simulink model "Querdynamikmodell"  (R2018b)
settings: Solver=VariableStepAuto  StartTime=0.0  StopTime=10.0  RelTol=1e-3
model workspace (MAT data in the model file):
  chStern = 20.5517740291
  controllerActive = 0
  cvStern = 205.517740291
  deltaH = [0 0.02 0.04 0.06 0.08 0.1 0.12 0.14 0.16 0.18 0.2 0.22 0.24 0.26 0.28 0.3 0.32 0.34 0.36 0.38 0.4 0.42 0.44 0.46 0.48 0.5 0.52 0.54 0.56 0.58 0.6 0.62 0.64 0.66 0.68 0.7 0.72 0.74 0.76 0.78 0.8 0.82 0.84 0.86 0.88 0.9 0.92 0.94 0.96 0.98 1 1.02 1.04 1.06 1.08 1.1 1.12 1.14 1.16 1.18 1.2 1.22 1.24 1.26 1.28 1.3 1.32 1.34 1.36 1.38 1.4 1.42 1.44 1.46 1.48 1.5 1.52 1.54 1.56 1.58 1.6 1.62 1.64 1.66 1.68 1.7 1.72 1.74 1.76 1.78 1.8 1.82 1.84 1.86 1.88 1.9 1.92 1.94 1.96 1.98 2 2.02 2.04 2.06 2.08 2.1 2.12 2.14 2.16 2.18 2.2 2.22 2.24 2.26 2.28 2.3 2.32 2.34 2.36 2.38 2.4 2.42 2.44 2.46 2.48 2.5 2.52 2.54 2.56 2.58 2.6 2.62 2.64 2.66 2.68 2.7 2.72 2.74 2.76 2.78 2.8 2.82 2.84 2.86 2.88 2.9 2.92 2.94 2.96 2.98 3 3.02 3.04 3.06 3.08 3.1 3.12 3.14 3.16 3.18 3.2 3.22 3.24 3.26 3.28 3.3 3.32 3.34 3.36 3.38 3.4 3.42 3.44 3.46 3.48 3.5 3.52 3.54 3.56 3.58 3.6 3.62 3.64 3.66 3.68 3.7 3.72 3.74 3.76 3.78 3.8 3.82 3.84 3.86 3.88 3.9 3.92 3.94 3.96 3.98 4 4.02 4.04 4.06 4.08 4.1 4.12 4.14 4.16 4.18 4.2 4.22 4.24 4.26 4.28 4.3 4.32 4.34 4.36 4.38 4.4 4.42 4.44 4.46 4.48 4.5 4.52 4.54 4.56 4.58 4.6 4.62 4.64 4.66 4.68 4.7 4.72 4.74 4.76 4.78 4.8 4.82 4.84 4.86 4.88 4.9 4.92 4.94 4.96 4.98 5 5.02 5.04 5.06 5.08 5.1 5.12 5.14 5.16 5.18 5.2 5.22 5.24 5.26 5.28 5.3 5.32 5.34 5.36 5.38 5.4 5.42 5.44 5.46 5.48 5.5 5.52 5.54 5.56 5.58 5.6 5.62 5.64 5.66 5.68 5.7 5.72 5.74 5.76 5.78 5.8 5.82 5.84 5.86 5.88 5.9 5.92 5.94 5.96 5.98 6]
  g = 9.81
  is = 16
  lh = 1.456
  lv = 1.344
  m = 1550
  r = 1
  theta = 2700
  v = 100
settings Model: Creator=gregoryseibert  LastModifiedBy=gregoryseibert

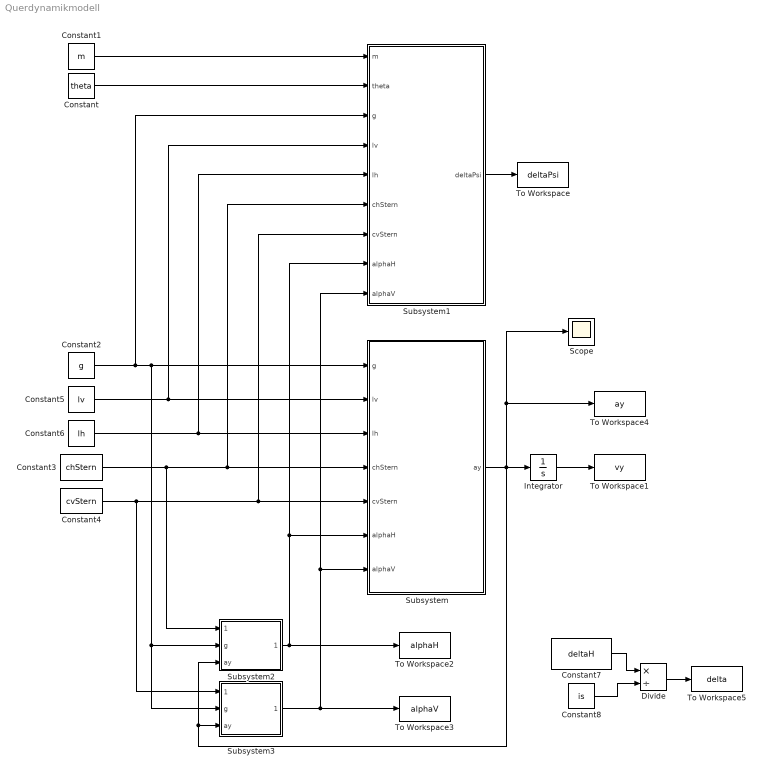
== system Querdynamikmodell ==
  Constant : Constant  Value=theta
  Constant1 : Constant  Value=m
  Constant2 : Constant  Value=g
  Constant3 : Constant  Value=chStern
  Constant4 : Constant  Value=cvStern
  Constant5 : Constant  Value=lv
  Constant6 : Constant  Value=lh
  Constant7 : Constant  Value=deltaH
  Constant8 : Constant  Value=is
  Divide : Product  Inputs=*/
  Integrator : Integrator
  Scope : Scope
  Subsystem : Subsystem
  Subsystem1 : Subsystem
  Subsystem2 : Subsystem
  Subsystem3 : Subsystem
  To Workspace : ToWorkspace  VariableName=deltaPsi  SaveFormat=Timeseries  SampleTime=-1
  To Workspace1 : ToWorkspace  VariableName=vy  SaveFormat=Timeseries  SampleTime=-1
  To Workspace2 : ToWorkspace  VariableName=alphaH  SaveFormat=Timeseries  SampleTime=-1
  To Workspace3 : ToWorkspace  VariableName=alphaV  SaveFormat=Timeseries  SampleTime=-1
  To Workspace4 : ToWorkspace  VariableName=ay  SaveFormat=Timeseries  SampleTime=-1
  To Workspace5 : ToWorkspace  VariableName=delta  SaveFormat=Timeseries  SampleTime=-1
  wires:
  Constant5/1 -> Subsystem1/4(lv), Subsystem/2(lv)
  Constant6/1 -> Subsystem/3(lh), Subsystem1/5(lh)
  Constant2/1 -> Subsystem3/2(g), Subsystem2/2(g), Subsystem/1(g), Subsystem1/3(g)
  Constant3/1 -> Subsystem2/1(chStern), Subsystem/4(chStern), Subsystem1/6(chStern)
  Constant4/1 -> Subsystem3/1(cvStern), Subsystem/5(cvStern), Subsystem1/7(cvStern)
  Subsystem/1(ay) -> Scope/1, To Workspace4/1, Subsystem2/3(ay), Subsystem3/3(ay), Integrator/1
  Constant1/1 -> Subsystem1/1(m)
  Constant/1 -> Subsystem1/2(theta)
  Subsystem1/1(deltaPsi) -> To Workspace/1
  Integrator/1 -> To Workspace1/1
  Subsystem2/1(alphaH) -> To Workspace2/1, Subsystem/6(alphaH), Subsystem1/8(alphaH)
  Subsystem3/1(alphaV) -> To Workspace3/1, Subsystem/7(alphaV), Subsystem1/9(alphaV)
  Constant7/1 -> Divide/1
  Constant8/1 -> Divide/2
  Divide/1 -> To Workspace5/1

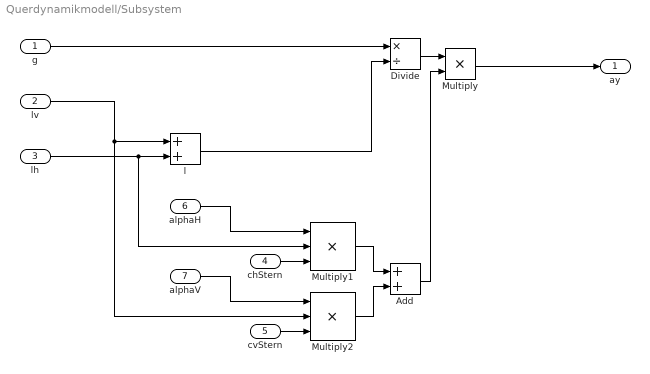
== system Querdynamikmodell/Subsystem ==
  g : Inport
  lv : Inport  Port=2
  lh : Inport  Port=3
  chStern : Inport  Port=4
  cvStern : Inport  Port=5
  alphaH : Inport  Port=6
  alphaV : Inport  Port=7
  Add : Sum
  Divide : Product  Inputs=*/
  Multiply : Product
  Multiply1 : Product  Inputs=3
  Multiply2 : Product  Inputs=3
  l : Sum
  ay : Outport
  wires:
  Multiply/1 -> ay/1
  g/1 -> Divide/1
  Divide/1 -> Multiply/1
  chStern/1 -> Multiply1/3
  alphaH/1 -> Multiply1/1
  Multiply2/1 -> Add/2
  l/1 -> Divide/2
  lv/1 -> Multiply2/2, l/1
  Multiply1/1 -> Add/1
  cvStern/1 -> Multiply2/3
  lh/1 -> Multiply1/2, l/2
  Add/1 -> Multiply/2
  alphaV/1 -> Multiply2/1

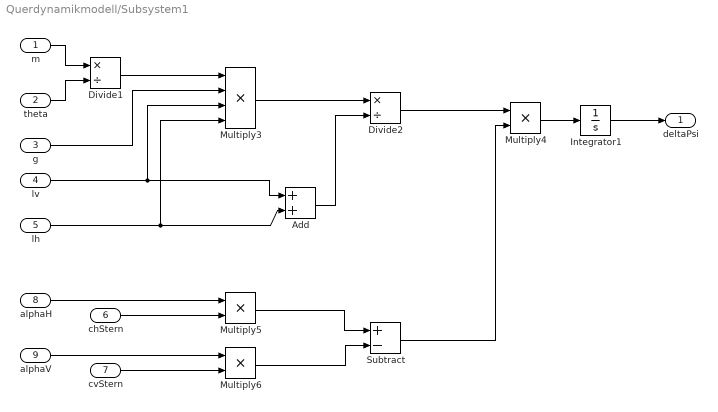
== system Querdynamikmodell/Subsystem1 ==
  m : Inport
  theta : Inport  Port=2
  g : Inport  Port=3
  lv : Inport  Port=4
  lh : Inport  Port=5
  chStern : Inport  Port=6
  cvStern : Inport  Port=7
  alphaH : Inport  Port=8
  alphaV : Inport  Port=9
  Add : Sum
  Divide1 : Product  Inputs=*/
  Divide2 : Product  Inputs=*/
  Integrator1 : Integrator
  Multiply3 : Product  Inputs=4
  Multiply4 : Product
  Multiply5 : Product
  Multiply6 : Product
  Subtract : Sum  Inputs=+-
  deltaPsi : Outport
  wires:
  Integrator1/1 -> deltaPsi/1
  theta/1 -> Divide1/2
  cvStern/1 -> Multiply6/2
  Multiply6/1 -> Subtract/2
  Add/1 -> Divide2/2
  Multiply4/1 -> Integrator1/1
  alphaH/1 -> Multiply5/1
  Divide1/1 -> Multiply3/1
  m/1 -> Divide1/1
  chStern/1 -> Multiply5/2
  Subtract/1 -> Multiply4/2
  Multiply3/1 -> Divide2/1
  Multiply5/1 -> Subtract/1
  Divide2/1 -> Multiply4/1
  g/1 -> Multiply3/2
  alphaV/1 -> Multiply6/1
  lv/1 -> Add/1, Multiply3/3
  lh/1 -> Multiply3/4, Add/2

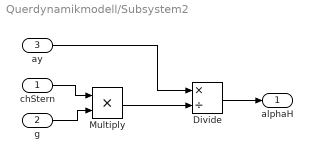
== system Querdynamikmodell/Subsystem2 ==
  chStern : Inport
  g : Inport  Port=2
  ay : Inport  Port=3
  Divide : Product  Inputs=*/
  Multiply : Product
  alphaH : Outport
  wires:
  g/1 -> Multiply/2
  chStern/1 -> Multiply/1
  ay/1 -> Divide/1
  Divide/1 -> alphaH/1
  Multiply/1 -> Divide/2

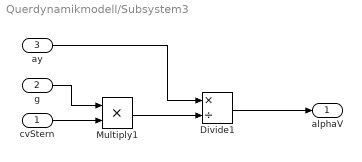
== system Querdynamikmodell/Subsystem3 ==
  cvStern : Inport
  g : Inport  Port=2
  ay : Inport  Port=3
  Divide1 : Product  Inputs=*/
  Multiply1 : Product
  alphaV : Outport
  wires:
  cvStern/1 -> Multiply1/2
  ay/1 -> Divide1/1
  g/1 -> Multiply1/1
  Divide1/1 -> alphaV/1
  Multiply1/1 -> Divide1/2
